simulink model "Buck_Boost"  (R2025a)
settings: Solver=VariableStepAuto  StartTime=0.0  StopTime=10.0  RelTol=1e-3  AbsTol=1e-3
libraries: fl_lib x6, nesl_utility x4, ee_lib x2
settings Model: Creator=daniel  LastModifiedBy=daniel
settings SolverCC: AutoScaleAbsTol=off  AlgebraicLoopSolver=TrustRegion  MaxZcPerStep=1.0
settings DebuggingCC: UnconnectedInputMsg=warning  UnconnectedOutputMsg=warning  UnconnectedLineMsg=warning  SymbolicDimsDataTypeCodeGenerationDiagnostic=none
settings ModelReferenceCC: EnableRefExpFcnMdlSchedulingChecks=on
settings SFSimCC: CustomCodeUndefinedFunction=UseInterfaceOnly
settings RTWCC: GPUComputeCapability=3.5  DLArmComputeVersion=19.05
settings SimscapeCC: SimscapeLogType=all  SimscapeLogSimulationStatistics=on  SimscapeLogDataHistory=10000.0

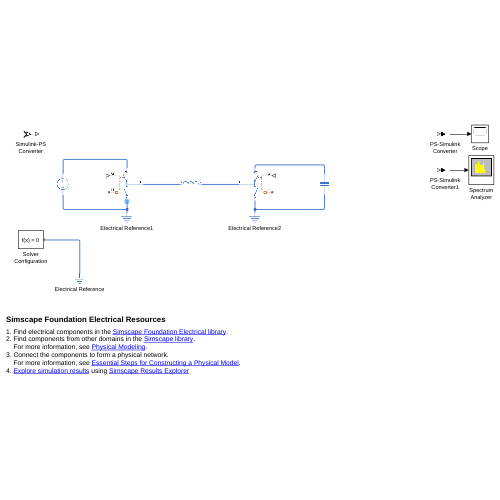
[thumbnail: Simulink's stored preview of the top-level diagram]
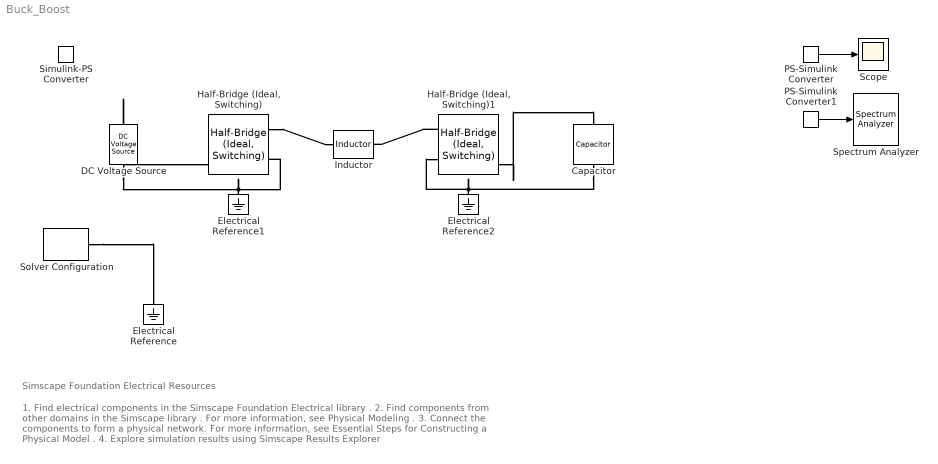
== system Buck_Boost ==
  note: 1. Find electrical components in the Simscape Foundation Electrical library .
      | 2. Find components from other domains in the Simscape library .
      | For more information, see Physical Modeling .
      | 3. Connect the components to form a physical network.
      | For more information, see Essential Steps for Constructing a Physical Model .
      | 4. Explore simulation results using Simscape Results Explorer
  note: Simscape Foundation Electrical Resources
  Capacitor : fl_lib/Electrical/Electrical Elements/Capacitor  c=30 uF  r=1e-6 Ohm  g=0 1/Ohm  i_specify=off  i_priority=None  i=0 A  i_nominal_specify=off  i_nominal_value=1  i_nominal_unit=A  v_specify=off  v_priority=None  v=0 V  v_nominal_specify=off  v_nominal_value=1  v_nominal_unit=V  vc_specify=off  vc_priority=High  vc=0 V  vc_nominal_specify=off  vc_nominal_value=1  vc_nominal_unit=V
  DC Voltage Source : fl_lib/Electrical/Electrical Sources/DC Voltage Source  v0=1 V
  Electrical Reference : fl_lib/Electrical/Electrical Elements/Electrical Reference
  Electrical Reference1 : fl_lib/Electrical/Electrical Elements/Electrical Reference
  Electrical Reference2 : fl_lib/Electrical/Electrical Elements/Electrical Reference
  "Half-Bridge (Ideal, Switching)" : ee_lib/Semiconductors & Converters/Half-Bridge (Ideal, Switching)  control_port=ee.enum.controlport.ps  device_type=ee.enum.converters.switches.mosfet  gto_Vgt=6 V  gto_Vgt_off=-1 V  gto_Ih=1 A  gto_thermal_loss_option=ee.enum.converters.thermalLossOption.constantvalues  gto_Vf=0.8 V  gto_Ron=0.001 Ohm  gto_Von_data=[0, .1, .6, .8, 1, 1.3, 1.6, 2, 2.4; 0, .1, .7, 1, 1.2, 1.5, 1.9, 2.4, 2.8] V  gto_Tj=[298.15, 398.15] K  gto_Iout_data=[0, .1, 1, 5, 10, 20, 40, 70, 100] A  igbt_Vth=6 V  igbt_thermal_loss_option=ee.enum.converters.thermalLossOption.constantvalues  igbt_Vf=0.8 V  igbt_Ron=0.001 Ohm  igbt_Von_data=[0, .1, .6, .8, 1, 1.3, 1.6, 2, 2.4; 0, .1, .7, 1, 1.2, 1.5, 1.9, 2.4, 2.8] V  igbt_Tj=[298.15, 398.15] K  igbt_Iout_data=[0, .1, 1, 5, 10, 20, 40, 70, 100] A  mosfet_Vth=2 V  mosfet_thermal_loss_option=ee.enum.converters.thermalLossOption.constantvalues  mosfet_Rds=0.01 Ohm  mosfet_Von_data=[0, 1.1, 1.3, 1.45, 1.75, 2.25, 2.7; 0, 1, 1.15, 1.35, 1.7, 2.35, 3] V  mosfet_Tj=[298.15, 398.15] K  mosfet_Iout_data=[0, 10, 50, 100, 200, 400, 600] A  Goff=1e-6 1/Ohm  gto_Eon_data=[0, .0024, .024, .12, .2, .48, 1.04, 2.16, 3.24; 0, .003, .03, .15, .25, .6, 1.3, 2.7, 4.05] * 1e-3 J  igbt_Eon_data=[0, .0024, .024, .12, .2, .48, 1.04, 2.16, 3.24; 0, .003, .03, .15, .25, .6, 1.3, 2.7, 4.05] * 1e-3 J  mosfet_Eon_data=[0, .29, 1.43, 2.86, 5.71, 13.14, 22.86; 0, .57, 2.63, 5.14, 10.29, 20.57, 30.29] * 1e-3 J  gto_Eoff_data=[0, .0007, .0066, .033, .066, .17, .33, .83, 1.5; 0, .001, .01, .05, .1, .25, .5, 1.2, 2.2] * 1e-3 J  igbt_Eoff_data=[0, .0007, .0066, .033, .066, .17, .33, .83, 1.5; 0, .001, .01, .05, .1, .25, .5, 1.2, 2.2] * 1e-3 J  mosfet_Eoff_data=[0, .21, 1.07, 2.14, 4.29, 9.86, 17.14; 0, .43, 1.97, 3.86, 7.71, 15.43, 22.71] * 1e-3 J  igbt_Eon_data_3D=[zeros(2, 9, 3)] J  mosfet_Eon_data_3D=[zeros(2, 7, 3)] J  igbt_Eoff_data_3D=[zeros(2, 9, 3)] J  mosfet_Eoff_data_3D=[zeros(2, 7, 3)] J  gto_Erec_data=[0, .0031, .021, .11, .21, .43, .99, 1.71, 3.078; 0, .0041, .043, .2, .39, .77, 1.54, 2.27, 4.08] * 1e-3 J  igbt_Erec_data=[0, .0031, .021, .11, .21, .43, .99, 1.71, 3.078; 0, .0041, .043, .2, .39, .77, 1.54, 2.27, 4.08] * 1e-3 J  mosfet_Erec_data=[0, .0031, .021, .11, .21, .43, .99; 0, .0041, .043, .2, .39, .77, 1.54] * 1e-3 J  gto_Tj_loss=[298.15, 398.15] K  igbt_Tj_loss=[298.15, 398.15] K  mosfet_Tj_loss=[298.15, 398.15] K  gto_Iout_data_loss=[0, .1, 1, 5, 10, 20, 40, 70, 100] A  igbt_Iout_data_loss=[0, .1, 1, 5, 10, 20, 40, 70, 100] A  mosfet_Iout_data_loss=[0, 10, 50, 100, 200, 400, 600] A  gto_Eon_scalar=22.86e-3 J  igbt_Eon_scalar=22.86e-3 J  mosfet_Eon_scalar=22.86e-3 J  gto_Eoff_scalar=17.14e-3 J  igbt_Eoff_scalar=17.14e-3 J  mosfet_Eoff_scalar=17.14e-3 J  gto_Erec_scalar=5.70e-3 J  igbt_Erec_scalar=5.70e-3 J  mosfet_Erec_scalar=5.70e-3 J  gto_Iout_scalar=600 A  igbt_Iout_scalar=600 A  mosfet_Iout_scalar=600 A  igbt_tabulateWithVce=false  mosfet_tabulateWithVds=false  igbt_Vce_loss=[0, 150, 300] V  mosfet_Vds_loss=[0, 150, 300] V  Voff=300 V  gto_Eoff_natural_commutation=10e-3 J  applySwLossToSupply=false  tauApplySwLoss=1e-3 s  diode_param=ee.enum.include.no  diode_ModelType=ee.enum.converters.diodeModelType.pwl  diode_TableType=ee.enum.diode.tableType.IfMat  diode_ReverseIVType=ee.enum.diode.diodeReverseIV.constant  diode_IfMat=[.07, .12, .19, 1.75, 4.24, 7.32, 11.2; .16, .3, .72, 2.14, 4.02, 6.35, 9.12] A  diode_VfMat=[.9, 1.15, 1.25, 1.5, 1.75, 2.17, 2.6, 2.85; .58, .68, .75, 1.1, 1.38, 1.77, 2.27, 2.7] V  diode_TjVec=[25, 125] degC  diode_VfVec=[.5, .7, .9, 1.3, 1.7, 2.1, 2.5] V  diode_IfVec=[.1, .2, .5, 1, 2, 4, 7, 10] A  diode_IrMat=[1e-06, 2e-06, 5e-06, 1e-05, 2.5e-05, 5e-05, .0001; 2e-06, 5e-06, 1e-05, 4e-05, 8e-05, .0002, .0005] A  diode_VrMat=[10, 100, 200, 250, 300, 325, 350; 10, 70, 160, 220, 270, 300, 320] V  diode_VrVec=[10, 20, 40, 50, 70, 80, 100] V  diode_IrVec=[1e-06, 2e-06, 5e-06, 1e-05, 2e-05, 5e-05, .0001] A  diode_Vf=0.8 V  diode_Ron=0.001 Ohm  diode_Goff=1e-5 1/Ohm  separateThermalPort=false  separateThermalPortsForDiodes=false  thermal_network_parameterization=ee.enum.thermalNetworkTopology.external  thermal_mass_parameterization=ee.enum.thermalNetwork.timeconstant  Rth=[.03, .2] K/W  Rth_Cauer=[.03, .1, .2] K/W  Rth_Foster=[.08, .14, .22, .16] K/W  thermal_mass=[3, 25] J/K  thermal_mass_Cauer=[3, 10, 25] J/K  thermal_mass_Foster=[.001, .005, .05, .5] J/K  thermal_time_constant=[.1, 5] s  thermal_time_constant_Cauer=[.1, 1, 5] s  thermal_time_constant_Foster=[7e-05, .0007, .01, .08] s  thermal_mass_initial_temperatures=[25, 25] degC  thermal_mass_initial_temperatures_Cauer=[25, 25, 25] degC  junction_thermal_mass=0.1 J/K  Tvec_initial_Foster=[25, 25, 25, 25] degC  RthDiode=[.03, .2] K/W  RthCauerDiode=[.03, .1, .2] K/W  RthFosterDiode=[.08, .14, .22, .16] K/W  ThermalMassDiode=[3, 25] J/K  ThermalMassCauerDiode=[3, 10, 25] J/K  ThermalMassFosterDiode=[.001, .005, .05, .5] J/K  ThermalTauDiode=[.1, 5] s  ThermalTauCauerDiode=[.1, 1, 5] s  ThermalTauFosterDiode=[7e-05, .0007, .01, .08] s  ThermalMassInitTempDiode=[25, 25] degC  ThermalMassInitTempCauerDiode=[25, 25, 25] degC  JunctionThermalMassDiode=0.1 J/K  TVecInitialFosterDiode=[25, 25, 25, 25] degC  junction_temperature_specify=off  junction_temperature_priority=None  junction_temperature=25 degC  junction_temperature_nominal_specify=off  junction_temperature_nominal_value=1  junction_temperature_nominal_unit=degC  upperSwitchTemp_specify=off  upperSwitchTemp_priority=None  upperSwitchTemp=25 degC  upperSwitchTemp_nominal_specify=off  upperSwitchTemp_nominal_value=1  upperSwitchTemp_nominal_unit=degC  lowerSwitchTemp_specify=off  lowerSwitchTemp_priority=None  lowerSwitchTemp=25 degC  lowerSwitchTemp_nominal_specify=off  lowerSwitchTemp_nominal_value=1  lowerSwitchTemp_nominal_unit=degC  upperDiodeTemp_specify=off  upperDiodeTemp_priority=None  upperDiodeTemp=25 degC  upperDiodeTemp_nominal_specify=off  upperDiodeTemp_nominal_value=1  upperDiodeTemp_nominal_unit=degC  lowerDiodeTemp_specify=off  lowerDiodeTemp_priority=None  lowerDiodeTemp=25 degC  lowerDiodeTemp_nominal_specify=off  lowerDiodeTemp_nominal_value=1  lowerDiodeTemp_nominal_unit=degC
      settings: InternalSimscapePortConfiguration="{\"Bottom\":[{\"id\":\"n\",\"label\":\"-\",\"type\":\"foundation.electrical.electrical\"}],\"Left\":[{\"id\":\"G\",\"label\":\"G\",\"type\":\"input\"},{\"id\":\"H\",\"label\":\"H\",\"type\":\"foundation.thermal.thermal\"}],\"Right\":[{\"id\":\"o\",\"label\":\"o\",\"type\":\"foundation.electrical.electrical\"}],\"Top\":[{\"id\":\"p\",\"label\":\"+\",\"type\":\"foundation.electrical.electrical\"}]}"
  "Half-Bridge (Ideal, Switching)1" : ee_lib/Semiconductors & Converters/Half-Bridge (Ideal, Switching)  control_port=ee.enum.controlport.ps  device_type=ee.enum.converters.switches.mosfet  gto_Vgt=6 V  gto_Vgt_off=-1 V  gto_Ih=1 A  gto_thermal_loss_option=ee.enum.converters.thermalLossOption.constantvalues  gto_Vf=0.8 V  gto_Ron=0.001 Ohm  gto_Von_data=[0, .1, .6, .8, 1, 1.3, 1.6, 2, 2.4; 0, .1, .7, 1, 1.2, 1.5, 1.9, 2.4, 2.8] V  gto_Tj=[298.15, 398.15] K  gto_Iout_data=[0, .1, 1, 5, 10, 20, 40, 70, 100] A  igbt_Vth=6 V  igbt_thermal_loss_option=ee.enum.converters.thermalLossOption.constantvalues  igbt_Vf=0.8 V  igbt_Ron=0.001 Ohm  igbt_Von_data=[0, .1, .6, .8, 1, 1.3, 1.6, 2, 2.4; 0, .1, .7, 1, 1.2, 1.5, 1.9, 2.4, 2.8] V  igbt_Tj=[298.15, 398.15] K  igbt_Iout_data=[0, .1, 1, 5, 10, 20, 40, 70, 100] A  mosfet_Vth=2 V  mosfet_thermal_loss_option=ee.enum.converters.thermalLossOption.constantvalues  mosfet_Rds=0.01 Ohm  mosfet_Von_data=[0, 1.1, 1.3, 1.45, 1.75, 2.25, 2.7; 0, 1, 1.15, 1.35, 1.7, 2.35, 3] V  mosfet_Tj=[298.15, 398.15] K  mosfet_Iout_data=[0, 10, 50, 100, 200, 400, 600] A  Goff=1e-6 1/Ohm  gto_Eon_data=[0, .0024, .024, .12, .2, .48, 1.04, 2.16, 3.24; 0, .003, .03, .15, .25, .6, 1.3, 2.7, 4.05] * 1e-3 J  igbt_Eon_data=[0, .0024, .024, .12, .2, .48, 1.04, 2.16, 3.24; 0, .003, .03, .15, .25, .6, 1.3, 2.7, 4.05] * 1e-3 J  mosfet_Eon_data=[0, .29, 1.43, 2.86, 5.71, 13.14, 22.86; 0, .57, 2.63, 5.14, 10.29, 20.57, 30.29] * 1e-3 J  gto_Eoff_data=[0, .0007, .0066, .033, .066, .17, .33, .83, 1.5; 0, .001, .01, .05, .1, .25, .5, 1.2, 2.2] * 1e-3 J  igbt_Eoff_data=[0, .0007, .0066, .033, .066, .17, .33, .83, 1.5; 0, .001, .01, .05, .1, .25, .5, 1.2, 2.2] * 1e-3 J  mosfet_Eoff_data=[0, .21, 1.07, 2.14, 4.29, 9.86, 17.14; 0, .43, 1.97, 3.86, 7.71, 15.43, 22.71] * 1e-3 J  igbt_Eon_data_3D=[zeros(2, 9, 3)] J  mosfet_Eon_data_3D=[zeros(2, 7, 3)] J  igbt_Eoff_data_3D=[zeros(2, 9, 3)] J  mosfet_Eoff_data_3D=[zeros(2, 7, 3)] J  gto_Erec_data=[0, .0031, .021, .11, .21, .43, .99, 1.71, 3.078; 0, .0041, .043, .2, .39, .77, 1.54, 2.27, 4.08] * 1e-3 J  igbt_Erec_data=[0, .0031, .021, .11, .21, .43, .99, 1.71, 3.078; 0, .0041, .043, .2, .39, .77, 1.54, 2.27, 4.08] * 1e-3 J  mosfet_Erec_data=[0, .0031, .021, .11, .21, .43, .99; 0, .0041, .043, .2, .39, .77, 1.54] * 1e-3 J  gto_Tj_loss=[298.15, 398.15] K  igbt_Tj_loss=[298.15, 398.15] K  mosfet_Tj_loss=[298.15, 398.15] K  gto_Iout_data_loss=[0, .1, 1, 5, 10, 20, 40, 70, 100] A  igbt_Iout_data_loss=[0, .1, 1, 5, 10, 20, 40, 70, 100] A  mosfet_Iout_data_loss=[0, 10, 50, 100, 200, 400, 600] A  gto_Eon_scalar=22.86e-3 J  igbt_Eon_scalar=22.86e-3 J  mosfet_Eon_scalar=22.86e-3 J  gto_Eoff_scalar=17.14e-3 J  igbt_Eoff_scalar=17.14e-3 J  mosfet_Eoff_scalar=17.14e-3 J  gto_Erec_scalar=5.70e-3 J  igbt_Erec_scalar=5.70e-3 J  mosfet_Erec_scalar=5.70e-3 J  gto_Iout_scalar=600 A  igbt_Iout_scalar=600 A  mosfet_Iout_scalar=600 A  igbt_tabulateWithVce=false  mosfet_tabulateWithVds=false  igbt_Vce_loss=[0, 150, 300] V  mosfet_Vds_loss=[0, 150, 300] V  Voff=300 V  gto_Eoff_natural_commutation=10e-3 J  applySwLossToSupply=false  tauApplySwLoss=1e-3 s  diode_param=ee.enum.include.no  diode_ModelType=ee.enum.converters.diodeModelType.pwl  diode_TableType=ee.enum.diode.tableType.IfMat  diode_ReverseIVType=ee.enum.diode.diodeReverseIV.constant  diode_IfMat=[.07, .12, .19, 1.75, 4.24, 7.32, 11.2; .16, .3, .72, 2.14, 4.02, 6.35, 9.12] A  diode_VfMat=[.9, 1.15, 1.25, 1.5, 1.75, 2.17, 2.6, 2.85; .58, .68, .75, 1.1, 1.38, 1.77, 2.27, 2.7] V  diode_TjVec=[25, 125] degC  diode_VfVec=[.5, .7, .9, 1.3, 1.7, 2.1, 2.5] V  diode_IfVec=[.1, .2, .5, 1, 2, 4, 7, 10] A  diode_IrMat=[1e-06, 2e-06, 5e-06, 1e-05, 2.5e-05, 5e-05, .0001; 2e-06, 5e-06, 1e-05, 4e-05, 8e-05, .0002, .0005] A  diode_VrMat=[10, 100, 200, 250, 300, 325, 350; 10, 70, 160, 220, 270, 300, 320] V  diode_VrVec=[10, 20, 40, 50, 70, 80, 100] V  diode_IrVec=[1e-06, 2e-06, 5e-06, 1e-05, 2e-05, 5e-05, .0001] A  diode_Vf=0.8 V  diode_Ron=0.001 Ohm  diode_Goff=1e-5 1/Ohm  separateThermalPort=false  separateThermalPortsForDiodes=false  thermal_network_parameterization=ee.enum.thermalNetworkTopology.external  thermal_mass_parameterization=ee.enum.thermalNetwork.timeconstant  Rth=[.03, .2] K/W  Rth_Cauer=[.03, .1, .2] K/W  Rth_Foster=[.08, .14, .22, .16] K/W  thermal_mass=[3, 25] J/K  thermal_mass_Cauer=[3, 10, 25] J/K  thermal_mass_Foster=[.001, .005, .05, .5] J/K  thermal_time_constant=[.1, 5] s  thermal_time_constant_Cauer=[.1, 1, 5] s  thermal_time_constant_Foster=[7e-05, .0007, .01, .08] s  thermal_mass_initial_temperatures=[25, 25] degC  thermal_mass_initial_temperatures_Cauer=[25, 25, 25] degC  junction_thermal_mass=0.1 J/K  Tvec_initial_Foster=[25, 25, 25, 25] degC  RthDiode=[.03, .2] K/W  RthCauerDiode=[.03, .1, .2] K/W  RthFosterDiode=[.08, .14, .22, .16] K/W  ThermalMassDiode=[3, 25] J/K  ThermalMassCauerDiode=[3, 10, 25] J/K  ThermalMassFosterDiode=[.001, .005, .05, .5] J/K  ThermalTauDiode=[.1, 5] s  ThermalTauCauerDiode=[.1, 1, 5] s  ThermalTauFosterDiode=[7e-05, .0007, .01, .08] s  ThermalMassInitTempDiode=[25, 25] degC  ThermalMassInitTempCauerDiode=[25, 25, 25] degC  JunctionThermalMassDiode=0.1 J/K  TVecInitialFosterDiode=[25, 25, 25, 25] degC  junction_temperature_specify=off  junction_temperature_priority=None  junction_temperature=25 degC  junction_temperature_nominal_specify=off  junction_temperature_nominal_value=1  junction_temperature_nominal_unit=degC  upperSwitchTemp_specify=off  upperSwitchTemp_priority=None  upperSwitchTemp=25 degC  upperSwitchTemp_nominal_specify=off  upperSwitchTemp_nominal_value=1  upperSwitchTemp_nominal_unit=degC  lowerSwitchTemp_specify=off  lowerSwitchTemp_priority=None  lowerSwitchTemp=25 degC  lowerSwitchTemp_nominal_specify=off  lowerSwitchTemp_nominal_value=1  lowerSwitchTemp_nominal_unit=degC  upperDiodeTemp_specify=off  upperDiodeTemp_priority=None  upperDiodeTemp=25 degC  upperDiodeTemp_nominal_specify=off  upperDiodeTemp_nominal_value=1  upperDiodeTemp_nominal_unit=degC  lowerDiodeTemp_specify=off  lowerDiodeTemp_priority=None  lowerDiodeTemp=25 degC  lowerDiodeTemp_nominal_specify=off  lowerDiodeTemp_nominal_value=1  lowerDiodeTemp_nominal_unit=degC
      settings: InternalSimscapePortConfiguration="{\"Bottom\":[{\"id\":\"n\",\"label\":\"-\",\"type\":\"foundation.electrical.electrical\"}],\"Left\":[{\"id\":\"G\",\"label\":\"G\",\"type\":\"input\"},{\"id\":\"H\",\"label\":\"H\",\"type\":\"foundation.thermal.thermal\"}],\"Right\":[{\"id\":\"o\",\"label\":\"o\",\"type\":\"foundation.electrical.electrical\"}],\"Top\":[{\"id\":\"p\",\"label\":\"+\",\"type\":\"foundation.electrical.electrical\"}]}"
  Inductor : fl_lib/Electrical/Electrical Elements/Inductor  l=10 uH  r=0 Ohm  g=1e-9 1/Ohm  i_specify=off  i_priority=None  i=0 A  i_nominal_specify=off  i_nominal_value=1  i_nominal_unit=A  v_specify=off  v_priority=None  v=0 V  v_nominal_specify=off  v_nominal_value=1  v_nominal_unit=V  i_L_specify=off  i_L_priority=High  i_L=0 A  i_L_nominal_specify=off  i_L_nominal_value=1  i_L_nominal_unit=A
  PS-Simulink Converter : nesl_utility/PS-Simulink Converter  PhysicalDomain=network_engine_domain  SubClassName=ps_output  LeftPortType=input  RightPortType=output  PseudoPeriodic=off  Frequencies=[]  VectorFormat=inherit  Unit=inherit  AffineConversion=off
  PS-Simulink Converter1 : nesl_utility/PS-Simulink Converter  PhysicalDomain=network_engine_domain  SubClassName=ps_output  LeftPortType=input  RightPortType=output  PseudoPeriodic=off  Frequencies=[]  VectorFormat=inherit  Unit=inherit  AffineConversion=off
  Scope : Scope
  Simulink-PS Converter : nesl_utility/Simulink-PS Converter  PhysicalDomain=network_engine_domain  SubClassName=ps_input  LeftPortType=input  RightPortType=output  PseudoPeriodic=off  Frequencies=[]  NoiseDistribution=none  NoiseParameters=[]  Unit=1  AffineConversion=off  FilteringAndDerivatives=provide  SimscapeFilterOrder=1  InputFilterTimeConstant=0.001  UdotUserProvided=0
  Solver Configuration : nesl_utility/Solver Configuration  PhysicalDomain=network_engine_domain  SubClassName=solver  LeftPortType=input  RightPortType=generic  Tones=[]  Harmonics=[]  SimulateNoise=off  Profile=off  UseLocalSampling=off  EnableSwitchedLinearOptims=on  FrequencyDomain=off  UseCCode=off  RelTol=0.001  AbsTol=1e-06  MinStep=1e-09  ToWorkspace=off  RevertToSquareIcSolve=off  NumHomotopyIterations=100  PhasorMode=off  PhasorModeNumHarmonics=1  ConsistencySolver=NEWTON_XTOL_AFTER_FTOL  IndexReductionMethod=DerivativeReplacement  DoDC=off  ResidualTolerance=1e-09  ConsistencyTolSource=GLOBAL  ConsistencyAbsTol=0.001  ConsistencyRelTol=0.001  ConsistencyTolFactor=0.001  UseLocalSolver=off  LocalSolverChoice=NE_BACKWARD_EULER_ADVANCER  ResolveIndetEquations=on  FunctionEvalNumThread=1  LocalSolverSampleTime=0.001  DoFixedCost=off  MaxNonlinIter=3  MaxModeIter=2  ComputeImpulses=off  ImpulseIterations=2  LinearAlgebra=auto  LinearAlgebraNumThread=0  EquationFormulation=NE_TIME_EF  DelaysMemoryBudget=1024  AutomaticFiltering=on  FilteringTimeConstant=0.001  PartitionStorageMethod=AS_NEEDED  PartitionMemoryBudget=1024  PartitionMethod=ROBUST  MultibodyUseLocalSolver=off  MultibodyLocalSolverChoice=ODE1  MultibodyLocalSolverSampleTime=0.001
  Spectrum Analyzer : SpectrumAnalyzer  Method=Welch  SampleRate=10e3  PlotAsTwoSidedSpectrum=off  AxesScalingNumUpdates=10  Span=10e3  StartFrequency=-5e3  StopFrequency=5e3  AveragingMethod=Running  ShowGrid=off  AllowFFTLengthLessThanSamplesPerUpdate=on  SegLen=128
  wires:
  PS-Simulink Converter/1 -> Scope/1
  PS-Simulink Converter1/1 -> Spectrum Analyzer/1
  connections:
  Solver Configuration/RConn1 -- Electrical Reference/LConn1
  "Half-Bridge (Ideal, Switching)"/RConn1 -- Inductor/LConn1
  "Half-Bridge (Ideal, Switching)1"/RConn1 -- Inductor/RConn1
  "Half-Bridge (Ideal, Switching)1"/LConn3 -- Capacitor/LConn1
  Capacitor/RConn1 -- Electrical Reference2/LConn1 -- "Half-Bridge (Ideal, Switching)1"/RConn2
  DC Voltage Source/LConn1 -- "Half-Bridge (Ideal, Switching)"/LConn3
  DC Voltage Source/RConn1 -- Electrical Reference1/LConn1 -- "Half-Bridge (Ideal, Switching)"/RConn2
